simulink model "Simulink_ejercicio_3"  (R2016b)
settings: Solver=VariableStepAuto  StartTime=0.0  StopTime=50  FixedStep=dt  RelTol=1e-3  EnableMultiTasking=on
values from neighbouring files (symbols this model uses):
  A = [-1.9311e-02  8.8157e+00 -3.2170e+01 -5.7499e-01 ... (first row only)    [ejercicio3.m]
  B = [ 1.7370e-01 -2.1499e-03 0.0000e+00 -1.7555e-01]'    [ejercicio3.m]
  C = [ 0.000000e+00 5.729578e+01 0.000000e+00 0.000000e+00 ... (first row only)    [ejercicio3.m]
  D = 0    [ejercicio3.m]
  delta_e_dot_lim = [-60 60]*pi/180    [ejercicio3.m]
  delta_e_lim = [-30 30]*pi/180    [ejercicio3.m]
  Kalfa = -0.5    [ejercicio3.m]
  Kq = -0.25    [ejercicio3.m]
  tau_a = 1/20.2    (= 0.049504950495)    [ejercicio3.m]
  tau_F = 0.1    [ejercicio3.m]
settings Model: Creator=Jairo  LastModifiedBy=mluser
settings DataIOCC: LimitDataPoints=on  SaveFormat=Array
settings OptimizationCC: LifeSpan=inf
settings DebuggingCC: SolverPrmCheckMsg=warning  SFUnexpectedBacktrackingDiag=warning  SFNoUnconditionalDefaultTransitionDiag=warning  SFExecutionAtInitializationDiag=none
settings HardwareCC: ProdBitPerPointer=32  ProdBitPerSizeT=32  ProdBitPerPtrDiffT=32  ProdLargestAtomicFloat=None  ProdIntDivRoundTo=Undefined  ProdEndianess=Unspecified  ProdWordSize=32  ProdHWDeviceType=32-bit Generic
settings ModelReferenceCC: PropagateSignalLabelsOutOfModel=off
settings GRTTargetCC: TargetLangStandard=C89/C90 (ANSI)
settings ConfigComp: CovMetricSettings=dw  CovSaveCumulativeToWorkspaceVar=on  CovSaveSingleToWorkspaceVar=on  CovExternalEMLEnable=off  CovSFcnEnable=off

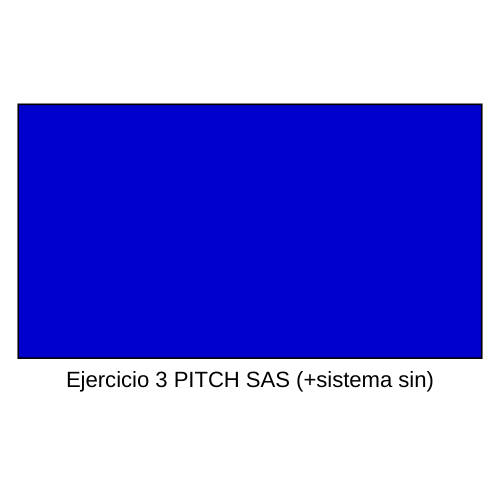
[thumbnail: Simulink's stored preview of the top-level diagram]
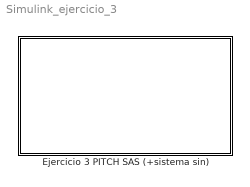
== system Simulink_ejercicio_3 ==
  Ejercicio 3 PITCH SAS (+sistema sin) : Subsystem

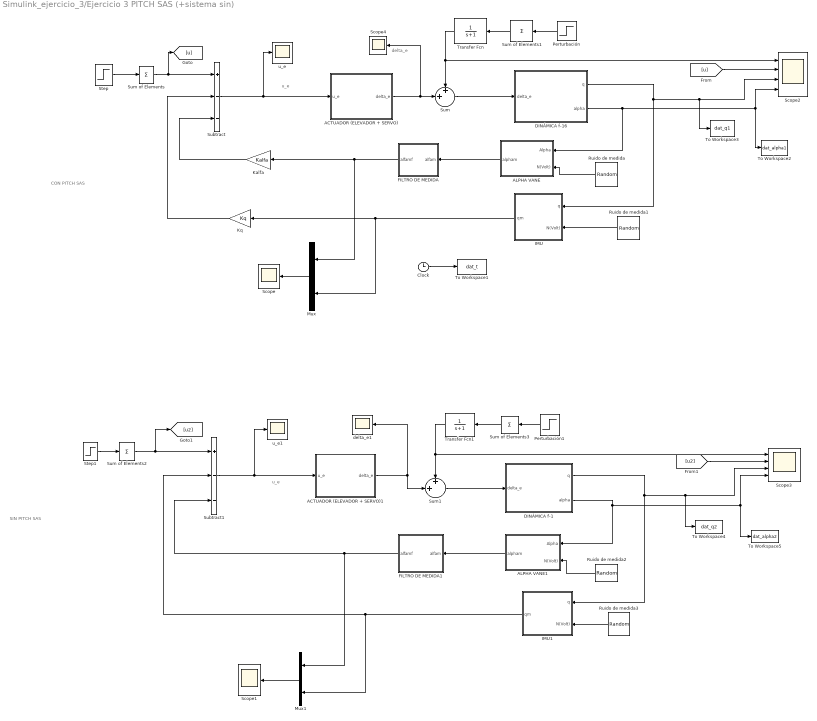
== system Simulink_ejercicio_3/Ejercicio 3 PITCH SAS (+sistema sin) ==
  note: delta_e
  note: u_e
  note: u_e
  note: SIN PITCH SAS
  note: CON PITCH SAS
  ACTUADOR (ELEVADOR + SERVO) : Subsystem
  ACTUADOR (ELEVADOR + SERVO)1 : Subsystem
  ALPHA VANE : Subsystem
  ALPHA VANE1 : Subsystem
  Clock : Clock
  DINÁMICA f-1 : Subsystem  mask(Dinámica F-16){A=A, B=B, C=C, D=D, Ci=[0 0 0 0]}
      mask prompts: A "Matriz de estados (A)"; B "Matriz de estados (B)"; C "Matriz de estados (C)"; D "Matriz de estados (D)"; Ci "Condiciones iniciales (nominales)"
  DINÁMICA f-16 : Subsystem  mask(Dinámica F-16){A=A, B=B, C=C, D=D, Ci=[0 0 0 0]}
      mask prompts: A "Matriz de estados (A)"; B "Matriz de estados (B)"; C "Matriz de estados (C)"; D "Matriz de estados (D)"; Ci "Condiciones iniciales (nominales)"
  FILTRO DE MEDIDA : Subsystem
  FILTRO DE MEDIDA1 : Subsystem
  IMU : Subsystem
  IMU1 : Subsystem
  Kalfa : Gain  Gain=Kalfa
  "Kq " : Gain  Gain=Kq
  Mux : Mux  Inputs=2
  Mux1 : Mux  Inputs=2
  Perturbación : Step  Time=[30 31]  Before=[0 0]  After=[-1 1]  SampleTime=0
  Perturbación1 : Step  Time=[30 31]  Before=[0 0]  After=[-1 1]  SampleTime=0
  Ruido de medida : RandomNumber  Variance=1e-4  Seed=123456  SampleTime=0.02
  Ruido de medida1 : RandomNumber  Variance=1e-5  Seed=123456  SampleTime=0.02
  Ruido de medida2 : RandomNumber  Variance=1e-4  Seed=123456  SampleTime=0.02
  Ruido de medida3 : RandomNumber  Variance=1e-5  Seed=123456  SampleTime=0.02
  Scope : Scope
  Scope1 : Scope
  Scope2 : Scope  NumInputPorts=4
  Scope3 : Scope  NumInputPorts=4
  Scope4 : Scope
  Step : Step  Time=[10 11]  Before=[0 0]  After=[1 -1]  SampleTime=0
  Step1 : Step  Time=[10 11]  Before=[0 0]  After=[1 -1]  SampleTime=0
  Subtract : Sum  Inputs=+--
  Subtract1 : Sum  Inputs=+--
  Sum : Sum  Inputs=++|  SaturateOnIntegerOverflow=on
  Sum of Elements{,1..3} (4 alike) : Sum  Inputs=+
  Sum1 : Sum  Inputs=++|  SaturateOnIntegerOverflow=on
  To Workspace1 : ToWorkspace  VariableName=dat_t  SampleTime=-1
  To Workspace2 : ToWorkspace  VariableName=dat_alpha1  SampleTime=-1
  To Workspace3 : ToWorkspace  VariableName=dat_q1  SampleTime=-1
  To Workspace4 : ToWorkspace  VariableName=dat_q2  SampleTime=-1
  To Workspace5 : ToWorkspace  VariableName=dat_alpha2  SampleTime=-1
  Transfer Fcn : TransferFcn  Denominator=[1 1]
  Transfer Fcn1 : TransferFcn  Denominator=[1 1]
  delta_e1 : Scope
  u_e : Scope
  u_e1 : Scope
  wires:
  IMU/1(qm) -> Mux/2, "Kq "/1
  DINÁMICA f-16/2(alpha) -> To Workspace2/1, Scope2/4, ALPHA VANE/1(Alpha)
  [u] -> Scope2/2
  Mux/1 -> Scope/1
  Sum of Elements1/1 -> Transfer Fcn/1
  Ruido de medida/1 -> ALPHA VANE/2(N(Volt))
  Ruido de medida1/1 -> IMU/2(N(Volt))
  Subtract/1 -> u_e/1, ACTUADOR (ELEVADOR + SERVO)/1(u_e)
  DINÁMICA f-16/1(q) -> IMU/1(q), To Workspace3/1, Scope2/3
  Sum/1 -> DINÁMICA f-16/1(delta_e)
  Step/1 -> Sum of Elements/1
  Perturbación/1 -> Sum of Elements1/1
  ACTUADOR (ELEVADOR + SERVO)/1(delta_e) -> Scope4/1, Sum/2
  "Kq "/1 -> Subtract/2
  Transfer Fcn/1 -> Sum/1, Scope2/1
  Kalfa/1 -> Subtract/3
  Sum of Elements/1 -> [u], Subtract/1
  ALPHA VANE/1(alpham) -> FILTRO DE MEDIDA/1(alfam)
  FILTRO DE MEDIDA/1(alfamf) -> Mux/1, Kalfa/1
  Clock/1 -> To Workspace1/1
  DINÁMICA f-1/2(alpha) -> To Workspace5/1, Scope3/4, ALPHA VANE1/1(Alpha)
  [u2] -> Scope3/2
  Mux1/1 -> Scope1/1
  Sum of Elements3/1 -> Transfer Fcn1/1
  Ruido de medida2/1 -> ALPHA VANE1/2(N(Volt))
  Ruido de medida3/1 -> IMU1/2(N(Volt))
  Subtract1/1 -> ACTUADOR (ELEVADOR + SERVO)1/1(u_e), u_e1/1
  DINÁMICA f-1/1(q) -> IMU1/1(q), To Workspace4/1, Scope3/3
  Sum1/1 -> DINÁMICA f-1/1(delta_e)
  Step1/1 -> Sum of Elements2/1
  Perturbación1/1 -> Sum of Elements3/1
  ACTUADOR (ELEVADOR + SERVO)1/1(delta_e) -> delta_e1/1, Sum1/2
  IMU1/1(qm) -> Mux1/2, Subtract1/2
  Transfer Fcn1/1 -> Sum1/1, Scope3/1
  FILTRO DE MEDIDA1/1(alfamf) -> Mux1/1, Subtract1/3
  Sum of Elements2/1 -> [u2], Subtract1/1
  ALPHA VANE1/1(alpham) -> FILTRO DE MEDIDA1/1(alfam)

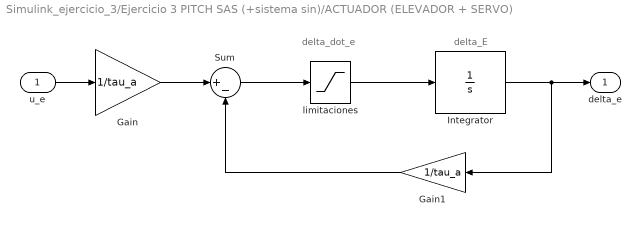
== system Simulink_ejercicio_3/Ejercicio 3 PITCH SAS (+sistema sin)/ACTUADOR (ELEVADOR + SERVO) ==
  note: delta_E
  note: delta_dot_e
  u_e : Inport
  Gain : Gain  Gain=1/tau_a
  Gain1 : Gain  Gain=1/tau_a
  Integrator : Integrator  LimitOutput=on  UpperSaturationLimit=delta_e_lim(2)  LowerSaturationLimit=delta_e_lim(1)
  Sum : Sum  Inputs=|+-
  limitaciones : Saturate  UpperLimit=delta_e_dot_lim(2)  LowerLimit=delta_e_dot_lim(1)
  delta_e : Outport
  wires:
  u_e/1 -> Gain/1
  Gain/1 -> Sum/1
  Sum/1 -> limitaciones/1
  limitaciones/1 -> Integrator/1
  Integrator/1 -> delta_e/1, Gain1/1
  Gain1/1 -> Sum/2

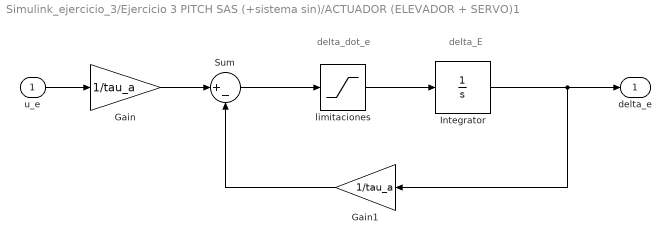
== system Simulink_ejercicio_3/Ejercicio 3 PITCH SAS (+sistema sin)/ACTUADOR (ELEVADOR + SERVO)1 ==
  note: delta_E
  note: delta_dot_e
  u_e : Inport
  Gain : Gain  Gain=1/tau_a
  Gain1 : Gain  Gain=1/tau_a
  Integrator : Integrator  LimitOutput=on  UpperSaturationLimit=delta_e_lim(2)  LowerSaturationLimit=delta_e_lim(1)
  Sum : Sum  Inputs=|+-
  limitaciones : Saturate  UpperLimit=delta_e_dot_lim(2)  LowerLimit=delta_e_dot_lim(1)
  delta_e : Outport
  wires:
  u_e/1 -> Gain/1
  Gain/1 -> Sum/1
  Sum/1 -> limitaciones/1
  limitaciones/1 -> Integrator/1
  Integrator/1 -> delta_e/1, Gain1/1
  Gain1/1 -> Sum/2

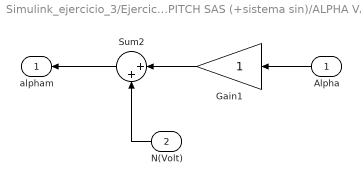
== system Simulink_ejercicio_3/Ejercicio 3 PITCH SAS (+sistema sin)/ALPHA VANE ==
  Alpha : Inport
  N(Volt) : Inport  Port=2
  Gain1 : Gain
  Sum2 : Sum  Inputs=|++
  alpham : Outport
  wires:
  Alpha/1 -> Gain1/1
  Gain1/1 -> Sum2/1
  N(Volt)/1 -> Sum2/2
  Sum2/1 -> alpham/1

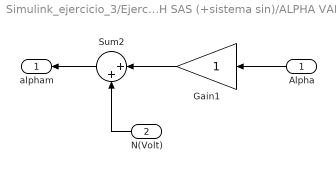
== system Simulink_ejercicio_3/Ejercicio 3 PITCH SAS (+sistema sin)/ALPHA VANE1 ==
  Alpha : Inport
  N(Volt) : Inport  Port=2
  Gain1 : Gain
  Sum2 : Sum  Inputs=|++
  alpham : Outport
  wires:
  Alpha/1 -> Gain1/1
  Gain1/1 -> Sum2/1
  N(Volt)/1 -> Sum2/2
  Sum2/1 -> alpham/1

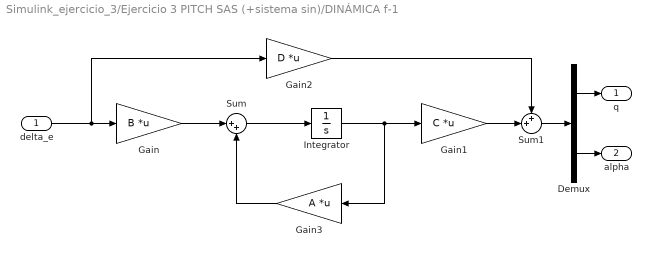
== system Simulink_ejercicio_3/Ejercicio 3 PITCH SAS (+sistema sin)/DINÁMICA f-1 ==
  delta_e : Inport
  Demux : Demux  Outputs=2
  Gain : Gain  Gain=B  Multiplication=Matrix(K*u)
  Gain1 : Gain  Gain=C  Multiplication=Matrix(K*u)
  Gain2 : Gain  Gain=D  Multiplication=Matrix(K*u)
  Gain3 : Gain  Gain=A  Multiplication=Matrix(K*u)
  Integrator : Integrator
  Sum : Sum  Inputs=|++
  Sum1 : Sum  Inputs=++|
  q : Outport
  alpha : Outport  Port=2
  wires:
  Gain/1 -> Sum/1
  Sum/1 -> Integrator/1
  Integrator/1 -> Gain3/1, Gain1/1
  delta_e/1 -> Gain2/1, Gain/1
  Gain2/1 -> Sum1/1
  Gain3/1 -> Sum/2
  Gain1/1 -> Sum1/2
  Demux/1 -> q/1
  Demux/2 -> alpha/1
  Sum1/1 -> Demux/1

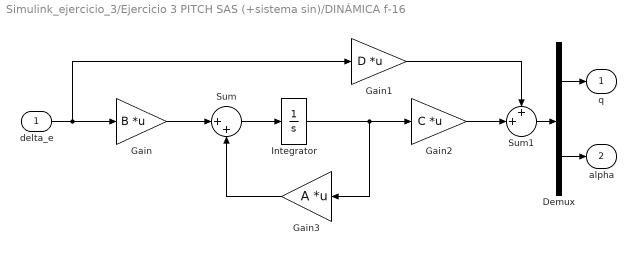
== system Simulink_ejercicio_3/Ejercicio 3 PITCH SAS (+sistema sin)/DINÁMICA f-16 ==
  delta_e : Inport
  Demux : Demux  Outputs=2
  Gain : Gain  Gain=B  Multiplication=Matrix(K*u)
  Gain1 : Gain  Gain=D  Multiplication=Matrix(K*u)
  Gain2 : Gain  Gain=C  Multiplication=Matrix(K*u)
  Gain3 : Gain  Gain=A  Multiplication=Matrix(K*u)
  Integrator : Integrator
  Sum : Sum  Inputs=|++
  Sum1 : Sum  Inputs=++|
  q : Outport
  alpha : Outport  Port=2
  wires:
  Gain/1 -> Sum/1
  Sum/1 -> Integrator/1
  Integrator/1 -> Gain3/1, Gain2/1
  delta_e/1 -> Gain1/1, Gain/1
  Gain1/1 -> Sum1/1
  Gain3/1 -> Sum/2
  Gain2/1 -> Sum1/2
  Demux/1 -> q/1
  Demux/2 -> alpha/1
  Sum1/1 -> Demux/1

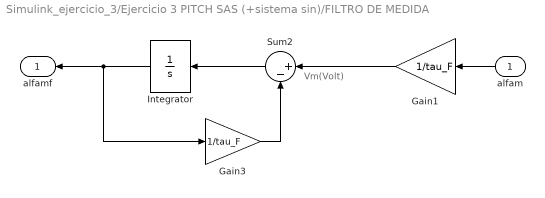
== system Simulink_ejercicio_3/Ejercicio 3 PITCH SAS (+sistema sin)/FILTRO DE MEDIDA ==
  note: Vm(Volt)
  alfam : Inport
  Gain1 : Gain  Gain=1/tau_F
  Gain3 : Gain  Gain=1/tau_F
  Integrator : Integrator
  Sum2 : Sum  Inputs=|+-
  alfamf : Outport
  wires:
  alfam/1 -> Gain1/1
  Gain1/1 -> Sum2/1
  Sum2/1 -> Integrator/1
  Gain3/1 -> Sum2/2
  Integrator/1 -> alfamf/1, Gain3/1

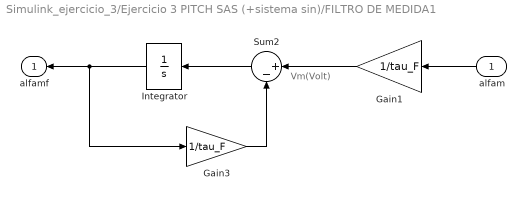
== system Simulink_ejercicio_3/Ejercicio 3 PITCH SAS (+sistema sin)/FILTRO DE MEDIDA1 ==
  note: Vm(Volt)
  alfam : Inport
  Gain1 : Gain  Gain=1/tau_F
  Gain3 : Gain  Gain=1/tau_F
  Integrator : Integrator
  Sum2 : Sum  Inputs=|+-
  alfamf : Outport
  wires:
  alfam/1 -> Gain1/1
  Gain1/1 -> Sum2/1
  Sum2/1 -> Integrator/1
  Gain3/1 -> Sum2/2
  Integrator/1 -> alfamf/1, Gain3/1

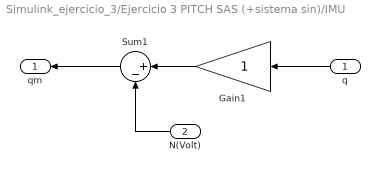
== system Simulink_ejercicio_3/Ejercicio 3 PITCH SAS (+sistema sin)/IMU ==
  q : Inport
  N(Volt) : Inport  Port=2
  Gain1 : Gain
  Sum1 : Sum  Inputs=|+-
  qm : Outport
  wires:
  q/1 -> Gain1/1
  Gain1/1 -> Sum1/1
  N(Volt)/1 -> Sum1/2
  Sum1/1 -> qm/1

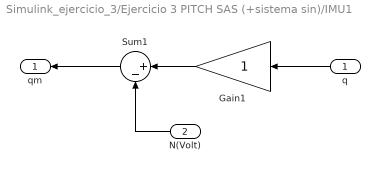
== system Simulink_ejercicio_3/Ejercicio 3 PITCH SAS (+sistema sin)/IMU1 ==
  q : Inport
  N(Volt) : Inport  Port=2
  Gain1 : Gain
  Sum1 : Sum  Inputs=|+-
  qm : Outport
  wires:
  q/1 -> Gain1/1
  Gain1/1 -> Sum1/1
  N(Volt)/1 -> Sum1/2
  Sum1/1 -> qm/1
